simulink model "Vehicle to vehicle major project BPMCE 2026 EEE"  (R2024b)
settings: Solver=FixedStepDiscrete  StartTime=0.0  StopTime=inf  FixedStep=0.05  RelTol=1e-3
libraries: slrealtimeiplib x1
settings Model: Creator=chand  LastModifiedBy=chand

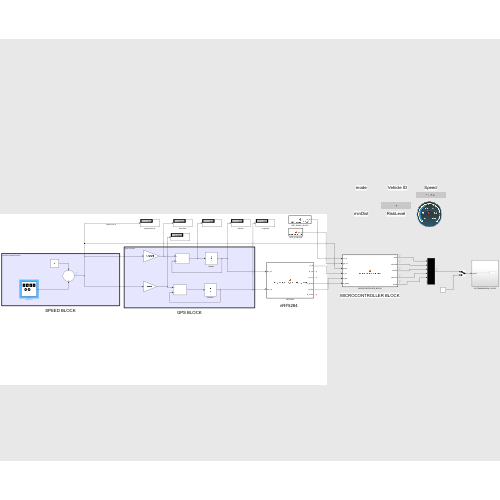
[thumbnail: Simulink's stored preview of the top-level diagram]
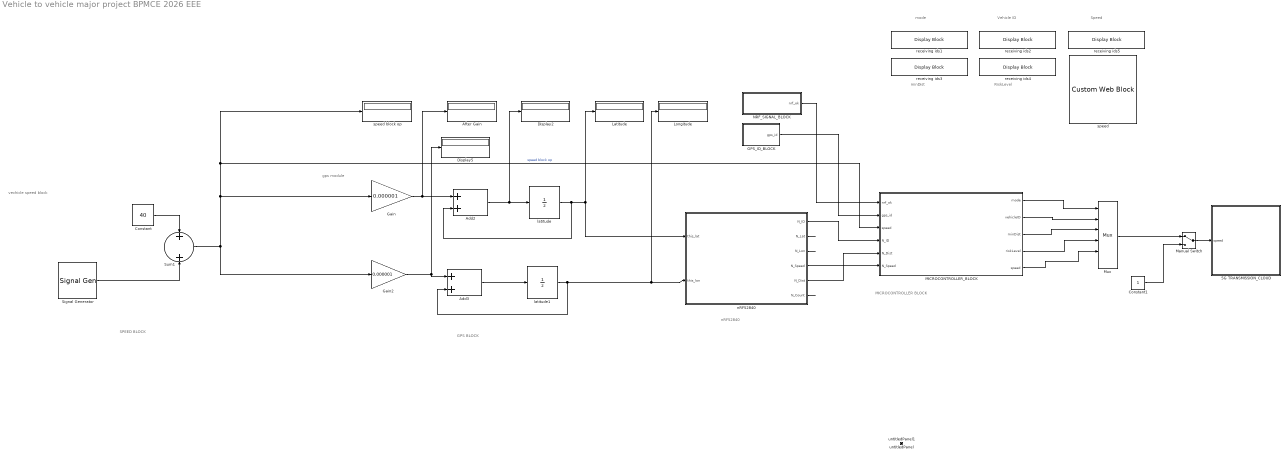
== system Vehicle to vehicle major project BPMCE 2026 EEE ==
  note: mode
  note: vechicle speed block
  note: gps module
  note: Vehicle ID
  note: minDist
  note: RiskLevel
  note: Speed
  note: GPS BLOCK
  note: SPEED BLOCK
  note: nRF52840
  note: MICROCONTROLLER BLOCK
  5G TRANSMISSION_CLOUD : Subsystem
  Add2 : Sum
  Add3 : Sum
  After Gain : Display
      settings: Decimation=5
  Constant : Constant  Value=40
  Constant1 : Constant
  Display2 : Display
  Display5 : Display
      settings: Decimation=5
  GPS_ID_BLOCK : MATLAB Function  TreatAsAtomicUnit=on
  Gain : Gain  Gain=0.000001
  Gain2 : Gain  Gain=0.000001
  Latitude : Display
  Longitude : Display
  MICROCONTROLLER_BLOCK : MATLAB Function  TreatAsAtomicUnit=on
  Manual Switch : ManualSwitch
  Mux : Mux  Inputs=6
  NRF_SIGNAL_BLOCK : MATLAB Function  TreatAsAtomicUnit=on
  Signal Generator : SignalGenerator  Amplitude=10  Units=rad/sec
  Sum1 : Sum
  latitude : UnitDelay  InitialCondition=25.900000  SampleTime=-1  HasFrameUpgradeWarning=on
  latitude1 : UnitDelay  InitialCondition=86.700000  SampleTime=-1  HasFrameUpgradeWarning=on
  nRF52840 : MATLAB Function  TreatAsAtomicUnit=on
  receiving ids{1..5} (5 alike) : DisplayBlock  LabelPosition=Hide  Transparency=1
  speed : CustomWebBlock  LabelPosition=Hide  ShowInitialText=on  Configuration="{\"components\":[{\"name\":\"CircularScaleComponent\",\"settings\":{\"bounds\":{\"max\":100,\"min\":0,\"tickInterval\":\"auto\"},\"direction\":\"cw\",\"flipLimits\":0,\"innerRadius\":0.75,\"internalTickHeightScaleFactor\":1,\"labelColor\":[255,255,200],\"labelFont\":{\"font\":\"Arial\",\"fontSize\":12},\"labelRadius\":0.528,\"labelTransparency\":1,\"minorTickHeightScaleFactor\":0.2,\"needleImage\":{\"size\":[200,50],\"src\":\"data:image\\/svg+xml;base64,PD94bWwgdmVyc2lvbj0iMS4wIiBlbmNvZGluZz0idXRmLTgiPz4KPCEtLSBHZW5lcmF0b3I6IEFkb2JlIElsbHVzdHJhdG9yIDI0LjEuMiwgU1ZHIEV4cG9ydCBQbHVnLUluIC4gU1ZHIFZlcnNpb246IDYuMDAgQnVpbGQgMCkgIC0tPgo8c3ZnIHZlcnNpb249IjEuMSIgaWQ9IkxheWVyXzEiIHhtbG5zPSJodHRwOi8vd3d3LnczLm9yZy8yMDAwL3N2ZyIgeG1sbnM6eGxpbms9Imh0dHA6Ly93d3cudzMub3JnLzE5OTkveGxpbmsiIHg9IjBweCIgeT0iMHB4IgoJIHZpZXdCb3g9IjAgMCAyMDAgNTAiIHN0eWxlPSJlbmFibGUtYmFja2dyb3VuZDpuZXcgMCAwIDIwMCA1MDsiIHhtbDpzcGFjZT0icHJlc2VydmUiPgo8c3R5bGUgdHlwZT0idGV4dC9jc3MiPgoJLnN0MHtmaWxsOiNFQzIxMjc7fQo8L3N0eWxlPgo8cGF0aCBjbGFzcz0ic3QwIiBkPSJNMTYyLjgsMTMuN0MxNjksNC40LDE4MS43LDEuOSwxOTEsOC4xczExLjgsMTguOSw1LjYsMjguMnMtMTguOSwxMS44LTI4LjIsNS42bDAsMAoJQzE1OS4xLDM1LjYsMTU2LjYsMjMsMTYyLjgsMTMuN0wxNjIuOCwxMy43eiBNMTY1LjgsMTUuOGMtNS4xLDcuNi0zLjEsMTcuOSw0LjYsMjNjNy42LDUuMSwxNy45LDMuMSwyMy00LjYKCWM1LjEtNy42LDMuMS0xNy45LTQuNi0yM2wwLDBDMTgxLjIsNi4yLDE3MC45LDguMiwxNjUuOCwxNS44eiIvPgo8cGF0aCBjbGFzcz0ic3QwIiBkPSJNMC40LDI1Ljl2LTMuM2wxNTktMi41Yy0wLjcsMi42LTAuNyw1LjIsMCw3LjhMMC40LDI1Ljl6Ii8+CjxjaXJjbGUgY2xhc3M9InN0MCIgY3g9IjE3OS42IiBjeT0iMjQiIHI9IjAuNyIvPgo8L3N2Zz4K\"},\"needleOffset\":[0.18464878250906522,0],\"needleOrientation\":-45,\"needleRotation\":180,\"needleSize\":{\"height\":0.11741692305346914,\"width\":0.46108337545091255},\"outerRadius\":0.9,\"position\":[0.05,0.05,0.9,0.9],\"referencePoint\":\"auto\",\"scaleAngle\":270,\"scaleAngleOffset\":135,\"scaleColors\":[],\"scaleColorsSize\":0.2,\"scaleDirection\":\"CW\",\"scalePosition\":[0,0,1,1],\"showLabels\":1,\"showMinorTicks\":1,\"showSpanLine\":1,\"showTicks\":1,\"tickColor\":[252,252,197],\"tickTransparency\":1,\"valueBarColor\":[0,114,189],\"valueBarPosition\":[0,0,1,1],\"valueBarSize\":0.2,\"valueBarTransparency\":1}},{\"name\":\"BackgroundImageComponent\",\"settings\":{\"image\":{\"size\":[500,500],\"src\":\"data:image\\/svg+xml;base64,PD94bWwgdmVyc2lvbj0iMS4wIiBlbmNvZGluZz0iVVRGLTgiIHN0YW5kYWxvbmU9Im5vIj8+CjxzdmcKICAgeG1sbnM6ZGM9Imh0dHA6Ly9wdXJsLm9yZy9kYy9lbGVtZW50cy8xLjEvIgogICB4bWxuczpjYz0iaHR0cDovL2NyZWF0aXZlY29tbW9ucy5vcmcvbnMjIgogICB4bWxuczpyZGY9Imh0dHA6Ly93d3cudzMub3JnLzE5OTkvMDIvMjItcmRmLXN5bnRheC1ucyMiCiAgIHhtbG5zOnN2Zz0iaHR0cDovL3d3dy53My5vcmcvMjAwMC9zdmciCiAgIHhtbG5zPSJodHRwOi8vd3d3LnczLm9yZy8yMDAwL3N2ZyIKICAgeG1sbnM6 ...(+9964 chars)\"},\"position\":[0,0,1,1],\"scaleMode\":\"0\"}},{\"name\":\"ForegroundImageComponent\",\"settings\":{\"image\":{\"size\":[0,0],\"src\":\"default\",\"srcOrientation\":[]},\"isForeground\":1,\"position\":[0,0,1,1],\"scaleMode\":\"0\"}}],\"settings\":{\"BindingType\":\"signal\",\"aspectRatio\":1.032258064516129,\"backgroundColor\":[0,0,0,\"1\"],\"backgroundOffset\":1,\"backgroundOpacity\":1,\"direction\":\"cw\",\"fixedAspectRatio\":\"on\",\"flipLimits\":0,\"orientation\":\"horizontal\",\"showBackgroundColor\":false,\"value\":0,\"version\":\"R2023a\"},\"type\":\"CircularGauge\"}"
  speed block op : Display
      settings: Decimation=5
  untitledPanel : Subsystem  Tag=HiddenForWebPanel  IsWebBlockPanel=on
  untitledPanel1 : Subsystem  Tag=HiddenForWebPanel  IsWebBlockPanel=on
  wires:
  Add3/1 -> latitude1/1
  Gain2/1 -> Add3/1, Display5/1
  Add2/1 -> latitude/1, Display2/1
  Gain/1 -> After Gain/1, Add2/1
  Constant/1 -> Sum1/1
  MICROCONTROLLER_BLOCK/5(speed) -> Mux/5
  nRF52840/4(N_Speed) -> MICROCONTROLLER_BLOCK/6(N_Speed)
  Sum1/1 -> Gain2/1, speed block op/1, MICROCONTROLLER_BLOCK/3("speed "), Gain/1  "speed block op"
  MICROCONTROLLER_BLOCK/3(minDist) -> Mux/3
  nRF52840/1(N_ID) -> MICROCONTROLLER_BLOCK/4(N_ID)
  MICROCONTROLLER_BLOCK/1(mode) -> Mux/1
  NRF_SIGNAL_BLOCK/1(nrf_ok) -> MICROCONTROLLER_BLOCK/1(nrf_ok)
  GPS_ID_BLOCK/1(gps_id) -> MICROCONTROLLER_BLOCK/2(gps_id)
  MICROCONTROLLER_BLOCK/4(riskLevel) -> Mux/4
  MICROCONTROLLER_BLOCK/2(vehicleID) -> Mux/2
  nRF52840/5(N_Dist) -> MICROCONTROLLER_BLOCK/5(N_Dist)
  latitude1/1 -> Longitude/1, nRF52840/2(this_lon), Add3/2
  latitude/1 -> nRF52840/1(this_lat), Latitude/1, Add2/2
  nRF52840/2(N_Lat) -> ?
  nRF52840/3(N_Lon) -> ?
  nRF52840/6(N_Count) -> ?
  Mux/1 -> Manual Switch/1
  Manual Switch/1 -> 5G TRANSMISSION_CLOUD/1(speed)
  Constant1/1 -> Manual Switch/2
  Signal Generator/1 -> Sum1/2

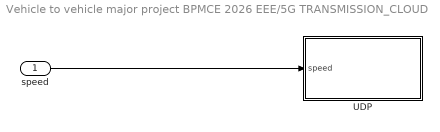
== system Vehicle to vehicle major project BPMCE 2026 EEE/5G TRANSMISSION_CLOUD ==
  speed : Inport
  UDP : Subsystem
  wires:
  speed/1 -> UDP/1(speed)

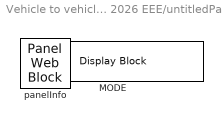
== system Vehicle to vehicle major project BPMCE 2026 EEE/untitledPanel ==
  MODE : DisplayBlock  Tag=HiddenForWebPanel  PanelInfo="{\"height\":40,\"left\":18,\"panelId\":\"panelId-3bc5ea36-2cb6-46e6-8433-6adb62cea3b6\",\"top\":18,\"type\":\"panelChild\",\"version\":\"2019b\",\"width\":180,\"zIndex\":1500002}"  LabelPosition=Hide  Transparency=1
  panelInfo : PanelWebBlock  Tag=HiddenForWebPanel  PanelInfo="{\"compacted\":false,\"height\":80,\"isActiveTab\":false,\"left\":409,\"name\":\"Panel\",\"panelId\":\"panelId-3bc5ea36-2cb6-46e6-8433-6adb62cea3b6\",\"popoutData\":{\"height\":206,\"left\":462,\"maximized\":false,\"top\":193,\"width\":236},\"popoutMode\":\"windowHidden\",\"tabIndex\":0,\"tabbedSetId\":\"tabbedSet0737036909\",\"top\":123,\"type\":\"panel\",\"version\":\"2019b\",\"visible\":false,\"width\":220,\"zIndex\":1500002}"  PanelSnapshot=<binary blob, 652 chars, not shown>

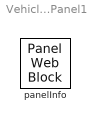
== system Vehicle to vehicle major project BPMCE 2026 EEE/untitledPanel1 ==
  panelInfo : PanelWebBlock  Tag=HiddenForWebPanel  PanelInfo="{\"compacted\":false,\"height\":80,\"isActiveTab\":true,\"left\":409,\"name\":\"Panel1\",\"panelId\":\"panelId-e718f758-56d7-42d4-b434-66c36aec679d\",\"popoutData\":{\"height\":206,\"left\":462,\"maximized\":false,\"top\":193,\"width\":236},\"popoutMode\":\"windowHidden\",\"tabIndex\":1,\"tabbedSetId\":\"tabbedSet0737036909\",\"top\":123,\"type\":\"panel\",\"version\":\"2019b\",\"visible\":true,\"width\":220,\"zIndex\":1499998}"  PanelSnapshot=<binary blob, 528 chars, not shown>

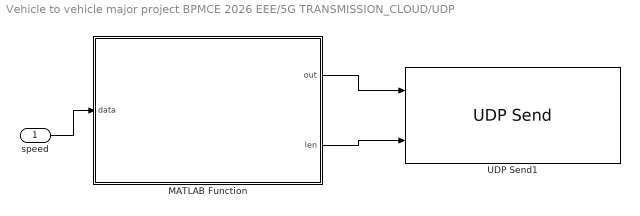
== system Vehicle to vehicle major project BPMCE 2026 EEE/5G TRANSMISSION_CLOUD/UDP ==
  speed : Inport
  MATLAB Function : MATLAB Function  TreatAsAtomicUnit=on
  UDP Send1 : slrealtimeiplib/UDP Send  useHostTargetConn=on  toAddress=127.0.0.1  toPort=4000  sampleTime=10  enableMessage=off
  wires:
  MATLAB Function/2(len) -> UDP Send1/2
  speed/1 -> MATLAB Function/1(data)
  MATLAB Function/1(out) -> UDP Send1/1

== matlab function Vehicle to vehicle major project BPMCE 2026 EEE/nRF52840 ==
  data: N_ID output; N_Lat output; N_Lon output; N_Speed output; N_Dist output; N_Count output; this_lat input; this_lon input
function [N_ID, N_Lat, N_Lon, N_Speed, N_Dist, N_Count] = ...
         NRF_MESH_BLOCK_RANDOM_40_FIXED(this_lat, this_lon)

maxN = 40;

persistent step

if isempty(step)
    step = 0;
end

step = step + 1;

% ---- Minimum distance oscillates between 5 and 20 m ----
minDist = 5 + mod(step, 16);   % 5 → 20 → 5 → ...

% ---- Fixed-size outputs ----
N_ID    = zeros(maxN,1);
N_Lat   = zeros(maxN,1);
N_Lon   = zeros(maxN,1);
N_Speed = zeros(maxN,1);
N_Dist  = zeros(maxN,1);

for i = 1:maxN
    % IDs look random but deterministic
    N_ID(i) = mod(i*17 + step*11, 200) + 1;

    % distances spread around minDist
    N_Dist(i) = minDist + mod(i*3, 25);  % some near, some far

    % fake GPS offset
    dlat = N_Dist(i) / 111000;
    N_Lat(i) = this_lat + dlat;
    N_Lon(i) = this_lon;

    % pseudo-random speed
    N_Speed(i) = 25 + mod(i*4 + step*3, 35);
end

% ---- Vehicles considered nearby (<= 50 m) ----
N_Count = sum(N_Dist <= 50);

== matlab function Vehicle to vehicle major project BPMCE 2026 EEE/5G TRANSMISSION_CLOUD/UDP/MATLAB Function ==
  data: data input; out output uint8 size=[1 200]; len output
function [out, len] = formatTelemetry(data)

MAX_LEN = 200;

mode      = data(1);
vehicleID = data(2);
minDist   = data(3);
riskLevel = data(4);
avgSpeed  = data(5);

str = sprintf( ...
'{"mode":%.0f,"vehicleID":%.0f,"minDist":%.2f,"riskLevel":%.0f,"avgSpeed":%.2f}', ...
mode, ...
vehicleID, ...
minDist, ...
riskLevel, ...
avgSpeed);

bytes = uint8(str);

len = length(bytes);

out = zeros(1, MAX_LEN, 'uint8');

out(1:len) = bytes;

end

== matlab function Vehicle to vehicle major project BPMCE 2026 EEE/MICROCONTROLLER_BLOCK ==
  data: nrf_ok input; gps_id input; mode output; vehicleID output; minDist output; riskLevel output; speed output; speed input; N_ID input; N_Dist input; N_Speed input
function [mode, vehicleID, minDist, riskLevel, speed] = ...
    MICROCONTROLLER_MAIN(nrf_ok, gps_id, speed, N_ID, N_Dist, N_Speed)

% -------- Persistent states --------
persistent minDist_p riskLevel_p vehicleID_p

if isempty(minDist_p)
    minDist_p = 0;
    riskLevel_p = 0;
    vehicleID_p = gps_id;
end

% -------- nRF WEAK → GPS ONLY --------
if nrf_ok == 0
    mode = 1;                  
    vehicleID = gps_id;        
    minDist = 0;               
    riskLevel = 0;
    return;
end

% -------- nRF OK → MESH MODE --------
mode = 0;

vehicleID_p = N_ID(1);         
minDist_p = min(N_Dist);

if minDist_p <= 8
    riskLevel_p = 3;
elseif minDist_p <= 12
    riskLevel_p = 2;
elseif minDist_p <= 18
    riskLevel_p = 1;
else
    riskLevel_p = 0;
end

vehicleID = vehicleID_p;
minDist   = minDist_p;
riskLevel = riskLevel_p;

end

== matlab function Vehicle to vehicle major project BPMCE 2026 EEE/NRF_SIGNAL_BLOCK ==
  data: nrf_ok output
function nrf_ok = NRF_SIGNAL_BLOCK
persistent c
if isempty(c)
    c = 0;
end
c = c + 1;

% 75% OK, 25% weak
if mod(c*7,100) < 75
    nrf_ok = 1;
else
    nrf_ok = 0;
end

== matlab function Vehicle to vehicle major project BPMCE 2026 EEE/GPS_ID_BLOCK ==
  data: gps_id output
function gps_id = GPS_ID_BLOCK
persistent id
if isempty(id)
    id = 1000;   % GPS-based ID range
end
gps_id = id;
